simulink model "TST_TClntDspl_DD"  (R2016b)
settings: Solver=FixedStepDiscrete  StartTime=0.0  StopTime=simTime  FixedStep=sampleTime  RelTol=1e-3
values from neighbouring files (symbols this model uses):
  testCase = 1    [initTST_TClntDspl_DD_001.m]    (also in initTST_TClntDspl_DD_002.m = 2; initTST_TClntDspl_DD_003.m = 3; initTST_TClntDspl_DD_004.m = 4; initTST_TClntDspl_DD_005.m = 5)
libraries: simulink x19, UnitTest_Lib x12
settings Model: Creator=liangyunbo  LastModifiedBy=liangyunbo
settings DebuggingCC: SignalRangeChecking=error

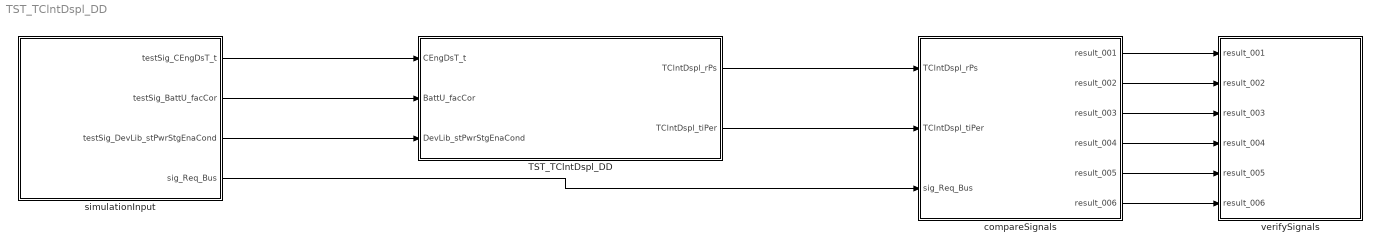
== system TST_TClntDspl_DD ==
  TST_TClntDspl_DD : Subsystem
  compareSignals : Subsystem
  simulationInput : Subsystem
  verifySignals : Subsystem
  wires:
  simulationInput/1(testSig_CEngDsT_t) -> TST_TClntDspl_DD/1(CEngDsT_t)
  simulationInput/2(testSig_BattU_facCor) -> TST_TClntDspl_DD/2(BattU_facCor)
  simulationInput/3(testSig_DevLib_stPwrStgEnaCond) -> TST_TClntDspl_DD/3(DevLib_stPwrStgEnaCond)
  TST_TClntDspl_DD/1(TClntDspl_rPs) -> compareSignals/1(TClntDspl_rPs)
  TST_TClntDspl_DD/2(TClntDspl_tiPer) -> compareSignals/2(TClntDspl_tiPer)
  simulationInput/4(sig_Req_Bus) -> compareSignals/3(sig_Req_Bus)
  compareSignals/1(result_001) -> verifySignals/1(result_001)
  compareSignals/2(result_002) -> verifySignals/2(result_002)
  compareSignals/3(result_003) -> verifySignals/3(result_003)
  compareSignals/4(result_004) -> verifySignals/4(result_004)
  compareSignals/5(result_005) -> verifySignals/5(result_005)
  compareSignals/6(result_006) -> verifySignals/6(result_006)

== system TST_TClntDspl_DD/TST_TClntDspl_DD ==
  CEngDsT_t : Inport
  BattU_facCor : Inport  Port=2
  DevLib_stPwrStgEnaCond : Inport  Port=3
  Function_Call : simulink/Ports & Subsystems/Function-Call Generator  sample_time=sampleTime  numberOfIterations=1
  TClntDspl_DD : ModelReference  ModelNameDialog=TClntDspl_DD  SimulationMode=Normal  ModelReferenceVersion=1.24  TriggerPortName=function  TriggerPortTriggerType=function-call  TriggerPortStatesWhenEnabling=held
  TClntDspl_rPs : Outport
  TClntDspl_tiPer : Outport  Port=2
  wires:
  Function_Call/1 -> TClntDspl_DD/Trigger
  CEngDsT_t/1 -> TClntDspl_DD/1
  BattU_facCor/1 -> TClntDspl_DD/2
  DevLib_stPwrStgEnaCond/1 -> TClntDspl_DD/3
  TClntDspl_DD/1 -> TClntDspl_rPs/1
  TClntDspl_DD/2 -> TClntDspl_tiPer/1

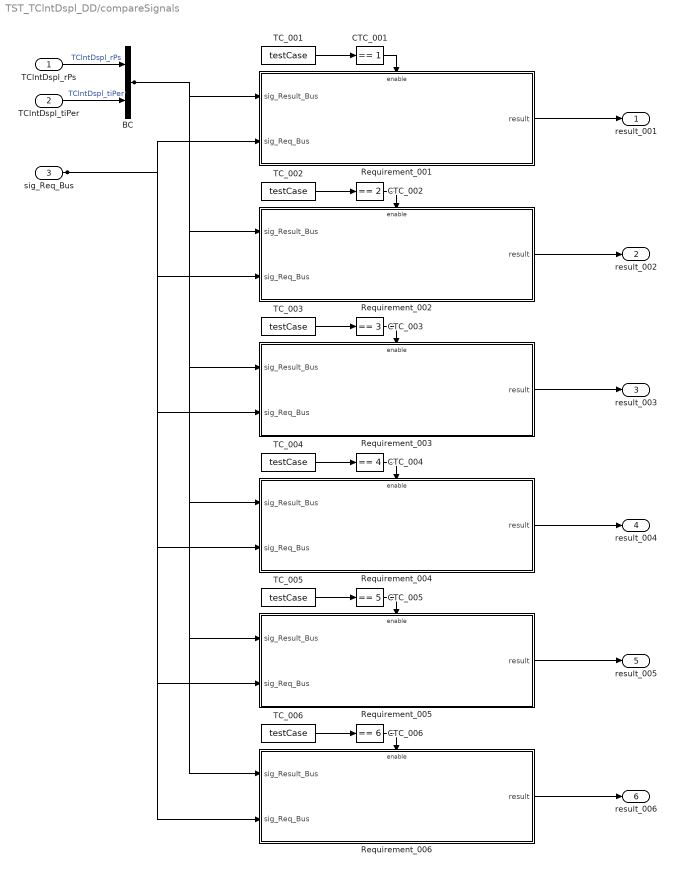
== system TST_TClntDspl_DD/compareSignals ==
  TClntDspl_rPs : Inport
  TClntDspl_tiPer : Inport  Port=2
  sig_Req_Bus : Inport  Port=3
  BC : BusCreator  Inputs=2
  CTC_001 : simulink/Logic and Bit Operations/Compare To Constant  relop===  const=1  OutDataTypeStr=boolean
  CTC_002 : simulink/Logic and Bit Operations/Compare To Constant  relop===  const=2  OutDataTypeStr=boolean
  CTC_003 : simulink/Logic and Bit Operations/Compare To Constant  relop===  const=3  OutDataTypeStr=boolean
  CTC_004 : simulink/Logic and Bit Operations/Compare To Constant  relop===  const=4  OutDataTypeStr=boolean
  CTC_005 : simulink/Logic and Bit Operations/Compare To Constant  relop===  const=5  OutDataTypeStr=boolean
  CTC_006 : simulink/Logic and Bit Operations/Compare To Constant  relop===  const=6  OutDataTypeStr=boolean
  Requirement_001 : Subsystem
  Requirement_002 : Subsystem
  Requirement_003 : Subsystem
  Requirement_004 : Subsystem
  Requirement_005 : Subsystem
  Requirement_006 : Subsystem
  TC_001 : Constant  Value=testCase
  TC_002 : Constant  Value=testCase
  TC_003 : Constant  Value=testCase
  TC_004 : Constant  Value=testCase
  TC_005 : Constant  Value=testCase
  TC_006 : Constant  Value=testCase
  result_001 : Outport
  result_002 : Outport  Port=2
  result_003 : Outport  Port=3
  result_004 : Outport  Port=4
  result_005 : Outport  Port=5
  result_006 : Outport  Port=6
  wires:
  TClntDspl_rPs/1 -> BC/1  "TClntDspl_rPs"
  TClntDspl_tiPer/1 -> BC/2  "TClntDspl_tiPer"
  TC_001/1 -> CTC_001/1
  CTC_001/1 -> Requirement_001/Enable
  sig_Req_Bus/1 -> Requirement_001/2(sig_Req_Bus), Requirement_002/2(sig_Req_Bus), Requirement_003/2(sig_Req_Bus), Requirement_004/2(sig_Req_Bus), Requirement_005/2(sig_Req_Bus), Requirement_006/2(sig_Req_Bus)
  BC/1 -> Requirement_001/1(sig_Result_Bus), Requirement_002/1(sig_Result_Bus), Requirement_003/1(sig_Result_Bus), Requirement_004/1(sig_Result_Bus), Requirement_005/1(sig_Result_Bus), Requirement_006/1(sig_Result_Bus)
  Requirement_001/1(result) -> result_001/1
  TC_002/1 -> CTC_002/1
  CTC_002/1 -> Requirement_002/Enable
  Requirement_002/1(result) -> result_002/1
  TC_003/1 -> CTC_003/1
  CTC_003/1 -> Requirement_003/Enable
  Requirement_003/1(result) -> result_003/1
  TC_004/1 -> CTC_004/1
  CTC_004/1 -> Requirement_004/Enable
  Requirement_004/1(result) -> result_004/1
  TC_005/1 -> CTC_005/1
  CTC_005/1 -> Requirement_005/Enable
  Requirement_005/1(result) -> result_005/1
  TC_006/1 -> CTC_006/1
  CTC_006/1 -> Requirement_006/Enable
  Requirement_006/1(result) -> result_006/1

== system TST_TClntDspl_DD/simulationInput ==
  BS : BusSelector  OutputSignals=testSig_CEngDsT_t,testSig_BattU_facCor,testSig_DevLib_stPwrStgEnaCond
  MPSw : MultiPortSwitch  Inputs=6  SaturateOnIntegerOverflow=on  InputSameDT=on
  TestCase : Constant  Value=testCase
  testSignals_R001 : Subsystem
  testSignals_R002 : Subsystem
  testSignals_R003 : Subsystem
  testSignals_R004 : Subsystem
  testSignals_R005 : Subsystem
  testSignals_R006 : Subsystem
  testSig_CEngDsT_t : Outport
  testSig_BattU_facCor : Outport  Port=2
  testSig_DevLib_stPwrStgEnaCond : Outport  Port=3
  sig_Req_Bus : Outport  Port=4
  wires:
  BS/1 -> testSig_CEngDsT_t/1  "<testSig_CEngDsT_t>"
  BS/2 -> testSig_BattU_facCor/1  "<testSig_BattU_facCor>"
  BS/3 -> testSig_DevLib_stPwrStgEnaCond/1  "<testSig_DevLib_stPwrStgEnaCond>"
  MPSw/1 -> BS/1, sig_Req_Bus/1
  TestCase/1 -> MPSw/1
  testSignals_R001/1(testSignals) -> MPSw/2
  testSignals_R002/1(testSignals) -> MPSw/3
  testSignals_R003/1(testSignals) -> MPSw/4
  testSignals_R004/1(testSignals) -> MPSw/5
  testSignals_R005/1(testSignals) -> MPSw/6
  testSignals_R006/1(testSignals) -> MPSw/7

== system TST_TClntDspl_DD/verifySignals ==
  result_001 : Inport
  result_002 : Inport  Port=2
  result_003 : Inport  Port=3
  result_004 : Inport  Port=4
  result_005 : Inport  Port=5
  result_006 : Inport  Port=6
  Assertion_001 : Assertion  Enabled=off
  Assertion_002 : Assertion  Enabled=off
  Assertion_003 : Assertion  Enabled=off
  Assertion_004 : Assertion  Enabled=off
  Assertion_005 : Assertion  Enabled=off
  Assertion_006 : Assertion  Enabled=off
  wires:
  result_001/1 -> Assertion_001/1
  result_002/1 -> Assertion_002/1
  result_003/1 -> Assertion_003/1
  result_004/1 -> Assertion_004/1
  result_005/1 -> Assertion_005/1
  result_006/1 -> Assertion_006/1

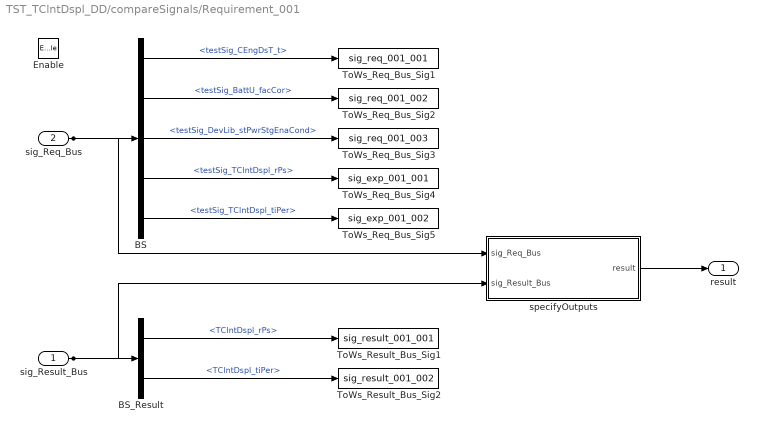
== system TST_TClntDspl_DD/compareSignals/Requirement_001 ==
  sig_Result_Bus : Inport
  sig_Req_Bus : Inport  Port=2
  Enable : EnablePort
  BS : BusSelector  OutputSignals=testSig_CEngDsT_t,testSig_BattU_facCor,testSig_DevLib_stPwrStgEnaCond,testSig_TClntDspl_rPs,testSig_TClntDspl_tiPer
  BS_Result : BusSelector  OutputSignals=TClntDspl_rPs,TClntDspl_tiPer
  ToWs_Req_Bus_Sig1 : ToWorkspace  VariableName=sig_req_001_001  SaveFormat=Structure With Time
  ToWs_Req_Bus_Sig2 : ToWorkspace  VariableName=sig_req_001_002  SaveFormat=Structure With Time
  ToWs_Req_Bus_Sig3 : ToWorkspace  VariableName=sig_req_001_003  SaveFormat=Structure With Time
  ToWs_Req_Bus_Sig4 : ToWorkspace  VariableName=sig_exp_001_001  SaveFormat=Structure With Time
  ToWs_Req_Bus_Sig5 : ToWorkspace  VariableName=sig_exp_001_002  SaveFormat=Structure With Time
  ToWs_Result_Bus_Sig1 : ToWorkspace  VariableName=sig_result_001_001  SaveFormat=Structure With Time
  ToWs_Result_Bus_Sig2 : ToWorkspace  VariableName=sig_result_001_002  SaveFormat=Structure With Time
  specifyOutputs : Subsystem
  result : Outport
  wires:
  sig_Req_Bus/1 -> BS/1, specifyOutputs/1(sig_Req_Bus)
  BS/1 -> ToWs_Req_Bus_Sig1/1  "<testSig_CEngDsT_t>"
  BS/2 -> ToWs_Req_Bus_Sig2/1  "<testSig_BattU_facCor>"
  BS/3 -> ToWs_Req_Bus_Sig3/1  "<testSig_DevLib_stPwrStgEnaCond>"
  BS/4 -> ToWs_Req_Bus_Sig4/1  "<testSig_TClntDspl_rPs>"
  BS/5 -> ToWs_Req_Bus_Sig5/1  "<testSig_TClntDspl_tiPer>"
  sig_Result_Bus/1 -> BS_Result/1, specifyOutputs/2(sig_Result_Bus)
  BS_Result/1 -> ToWs_Result_Bus_Sig1/1  "<TClntDspl_rPs>"
  BS_Result/2 -> ToWs_Result_Bus_Sig2/1  "<TClntDspl_tiPer>"
  specifyOutputs/1(result) -> result/1

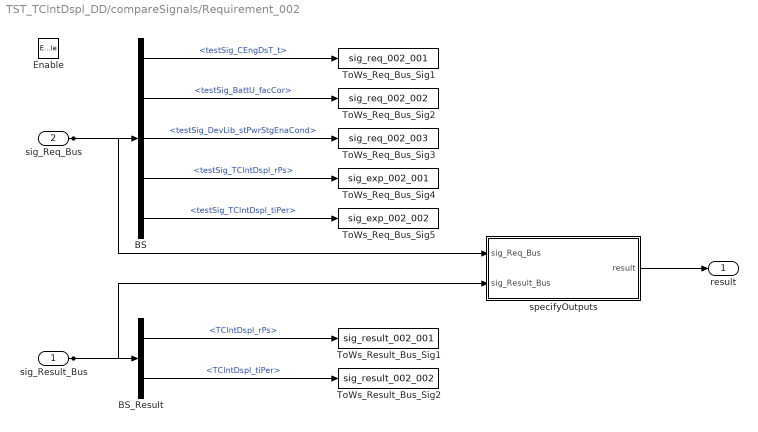
== system TST_TClntDspl_DD/compareSignals/Requirement_002 ==
  sig_Result_Bus : Inport
  sig_Req_Bus : Inport  Port=2
  Enable : EnablePort
  BS : BusSelector  OutputSignals=testSig_CEngDsT_t,testSig_BattU_facCor,testSig_DevLib_stPwrStgEnaCond,testSig_TClntDspl_rPs,testSig_TClntDspl_tiPer
  BS_Result : BusSelector  OutputSignals=TClntDspl_rPs,TClntDspl_tiPer
  ToWs_Req_Bus_Sig1 : ToWorkspace  VariableName=sig_req_002_001  SaveFormat=Structure With Time
  ToWs_Req_Bus_Sig2 : ToWorkspace  VariableName=sig_req_002_002  SaveFormat=Structure With Time
  ToWs_Req_Bus_Sig3 : ToWorkspace  VariableName=sig_req_002_003  SaveFormat=Structure With Time
  ToWs_Req_Bus_Sig4 : ToWorkspace  VariableName=sig_exp_002_001  SaveFormat=Structure With Time
  ToWs_Req_Bus_Sig5 : ToWorkspace  VariableName=sig_exp_002_002  SaveFormat=Structure With Time
  ToWs_Result_Bus_Sig1 : ToWorkspace  VariableName=sig_result_002_001  SaveFormat=Structure With Time
  ToWs_Result_Bus_Sig2 : ToWorkspace  VariableName=sig_result_002_002  SaveFormat=Structure With Time
  specifyOutputs : Subsystem
  result : Outport
  wires:
  sig_Req_Bus/1 -> BS/1, specifyOutputs/1(sig_Req_Bus)
  BS/1 -> ToWs_Req_Bus_Sig1/1  "<testSig_CEngDsT_t>"
  BS/2 -> ToWs_Req_Bus_Sig2/1  "<testSig_BattU_facCor>"
  BS/3 -> ToWs_Req_Bus_Sig3/1  "<testSig_DevLib_stPwrStgEnaCond>"
  BS/4 -> ToWs_Req_Bus_Sig4/1  "<testSig_TClntDspl_rPs>"
  BS/5 -> ToWs_Req_Bus_Sig5/1  "<testSig_TClntDspl_tiPer>"
  sig_Result_Bus/1 -> BS_Result/1, specifyOutputs/2(sig_Result_Bus)
  BS_Result/1 -> ToWs_Result_Bus_Sig1/1  "<TClntDspl_rPs>"
  BS_Result/2 -> ToWs_Result_Bus_Sig2/1  "<TClntDspl_tiPer>"
  specifyOutputs/1(result) -> result/1

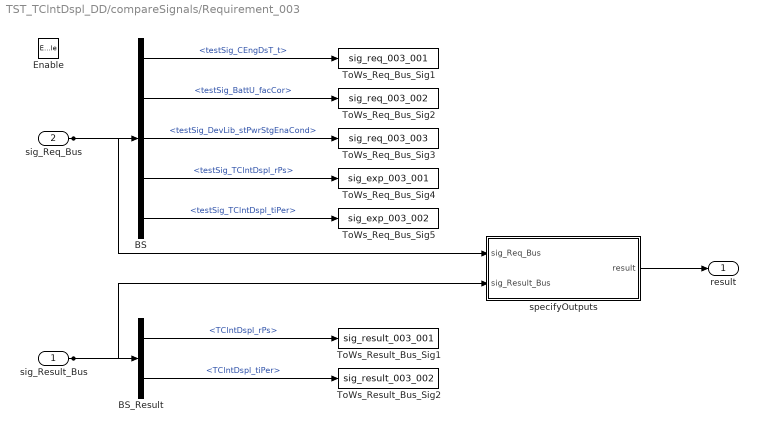
== system TST_TClntDspl_DD/compareSignals/Requirement_003 ==
  sig_Result_Bus : Inport
  sig_Req_Bus : Inport  Port=2
  Enable : EnablePort
  BS : BusSelector  OutputSignals=testSig_CEngDsT_t,testSig_BattU_facCor,testSig_DevLib_stPwrStgEnaCond,testSig_TClntDspl_rPs,testSig_TClntDspl_tiPer
  BS_Result : BusSelector  OutputSignals=TClntDspl_rPs,TClntDspl_tiPer
  ToWs_Req_Bus_Sig1 : ToWorkspace  VariableName=sig_req_003_001  SaveFormat=Structure With Time
  ToWs_Req_Bus_Sig2 : ToWorkspace  VariableName=sig_req_003_002  SaveFormat=Structure With Time
  ToWs_Req_Bus_Sig3 : ToWorkspace  VariableName=sig_req_003_003  SaveFormat=Structure With Time
  ToWs_Req_Bus_Sig4 : ToWorkspace  VariableName=sig_exp_003_001  SaveFormat=Structure With Time
  ToWs_Req_Bus_Sig5 : ToWorkspace  VariableName=sig_exp_003_002  SaveFormat=Structure With Time
  ToWs_Result_Bus_Sig1 : ToWorkspace  VariableName=sig_result_003_001  SaveFormat=Structure With Time
  ToWs_Result_Bus_Sig2 : ToWorkspace  VariableName=sig_result_003_002  SaveFormat=Structure With Time
  specifyOutputs : Subsystem
  result : Outport
  wires:
  sig_Req_Bus/1 -> BS/1, specifyOutputs/1(sig_Req_Bus)
  BS/1 -> ToWs_Req_Bus_Sig1/1  "<testSig_CEngDsT_t>"
  BS/2 -> ToWs_Req_Bus_Sig2/1  "<testSig_BattU_facCor>"
  BS/3 -> ToWs_Req_Bus_Sig3/1  "<testSig_DevLib_stPwrStgEnaCond>"
  BS/4 -> ToWs_Req_Bus_Sig4/1  "<testSig_TClntDspl_rPs>"
  BS/5 -> ToWs_Req_Bus_Sig5/1  "<testSig_TClntDspl_tiPer>"
  sig_Result_Bus/1 -> BS_Result/1, specifyOutputs/2(sig_Result_Bus)
  BS_Result/1 -> ToWs_Result_Bus_Sig1/1  "<TClntDspl_rPs>"
  BS_Result/2 -> ToWs_Result_Bus_Sig2/1  "<TClntDspl_tiPer>"
  specifyOutputs/1(result) -> result/1

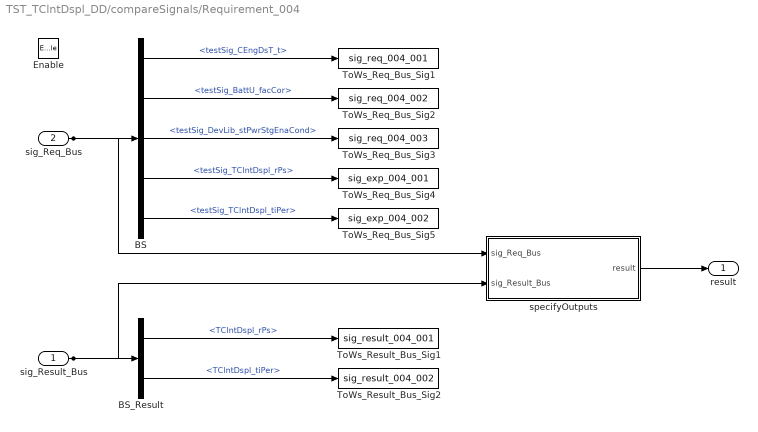
== system TST_TClntDspl_DD/compareSignals/Requirement_004 ==
  sig_Result_Bus : Inport
  sig_Req_Bus : Inport  Port=2
  Enable : EnablePort
  BS : BusSelector  OutputSignals=testSig_CEngDsT_t,testSig_BattU_facCor,testSig_DevLib_stPwrStgEnaCond,testSig_TClntDspl_rPs,testSig_TClntDspl_tiPer
  BS_Result : BusSelector  OutputSignals=TClntDspl_rPs,TClntDspl_tiPer
  ToWs_Req_Bus_Sig1 : ToWorkspace  VariableName=sig_req_004_001  SaveFormat=Structure With Time
  ToWs_Req_Bus_Sig2 : ToWorkspace  VariableName=sig_req_004_002  SaveFormat=Structure With Time
  ToWs_Req_Bus_Sig3 : ToWorkspace  VariableName=sig_req_004_003  SaveFormat=Structure With Time
  ToWs_Req_Bus_Sig4 : ToWorkspace  VariableName=sig_exp_004_001  SaveFormat=Structure With Time
  ToWs_Req_Bus_Sig5 : ToWorkspace  VariableName=sig_exp_004_002  SaveFormat=Structure With Time
  ToWs_Result_Bus_Sig1 : ToWorkspace  VariableName=sig_result_004_001  SaveFormat=Structure With Time
  ToWs_Result_Bus_Sig2 : ToWorkspace  VariableName=sig_result_004_002  SaveFormat=Structure With Time
  specifyOutputs : Subsystem
  result : Outport
  wires:
  sig_Req_Bus/1 -> BS/1, specifyOutputs/1(sig_Req_Bus)
  BS/1 -> ToWs_Req_Bus_Sig1/1  "<testSig_CEngDsT_t>"
  BS/2 -> ToWs_Req_Bus_Sig2/1  "<testSig_BattU_facCor>"
  BS/3 -> ToWs_Req_Bus_Sig3/1  "<testSig_DevLib_stPwrStgEnaCond>"
  BS/4 -> ToWs_Req_Bus_Sig4/1  "<testSig_TClntDspl_rPs>"
  BS/5 -> ToWs_Req_Bus_Sig5/1  "<testSig_TClntDspl_tiPer>"
  sig_Result_Bus/1 -> BS_Result/1, specifyOutputs/2(sig_Result_Bus)
  BS_Result/1 -> ToWs_Result_Bus_Sig1/1  "<TClntDspl_rPs>"
  BS_Result/2 -> ToWs_Result_Bus_Sig2/1  "<TClntDspl_tiPer>"
  specifyOutputs/1(result) -> result/1

== system TST_TClntDspl_DD/compareSignals/Requirement_005 ==
  sig_Result_Bus : Inport
  sig_Req_Bus : Inport  Port=2
  Enable : EnablePort
  BS : BusSelector  OutputSignals=testSig_CEngDsT_t,testSig_BattU_facCor,testSig_DevLib_stPwrStgEnaCond,testSig_TClntDspl_rPs,testSig_TClntDspl_tiPer
  BS_Result : BusSelector  OutputSignals=TClntDspl_rPs,TClntDspl_tiPer
  ToWs_Req_Bus_Sig1 : ToWorkspace  VariableName=sig_req_005_001  SaveFormat=Structure With Time
  ToWs_Req_Bus_Sig2 : ToWorkspace  VariableName=sig_req_005_002  SaveFormat=Structure With Time
  ToWs_Req_Bus_Sig3 : ToWorkspace  VariableName=sig_req_005_003  SaveFormat=Structure With Time
  ToWs_Req_Bus_Sig4 : ToWorkspace  VariableName=sig_exp_005_001  SaveFormat=Structure With Time
  ToWs_Req_Bus_Sig5 : ToWorkspace  VariableName=sig_exp_005_002  SaveFormat=Structure With Time
  ToWs_Result_Bus_Sig1 : ToWorkspace  VariableName=sig_result_005_001  SaveFormat=Structure With Time
  ToWs_Result_Bus_Sig2 : ToWorkspace  VariableName=sig_result_005_002  SaveFormat=Structure With Time
  specifyOutputs : Subsystem
  result : Outport
  wires:
  sig_Req_Bus/1 -> BS/1, specifyOutputs/1(sig_Req_Bus)
  BS/1 -> ToWs_Req_Bus_Sig1/1  "<testSig_CEngDsT_t>"
  BS/2 -> ToWs_Req_Bus_Sig2/1  "<testSig_BattU_facCor>"
  BS/3 -> ToWs_Req_Bus_Sig3/1  "<testSig_DevLib_stPwrStgEnaCond>"
  BS/4 -> ToWs_Req_Bus_Sig4/1  "<testSig_TClntDspl_rPs>"
  BS/5 -> ToWs_Req_Bus_Sig5/1  "<testSig_TClntDspl_tiPer>"
  sig_Result_Bus/1 -> BS_Result/1, specifyOutputs/2(sig_Result_Bus)
  BS_Result/1 -> ToWs_Result_Bus_Sig1/1  "<TClntDspl_rPs>"
  BS_Result/2 -> ToWs_Result_Bus_Sig2/1  "<TClntDspl_tiPer>"
  specifyOutputs/1(result) -> result/1

== system TST_TClntDspl_DD/compareSignals/Requirement_006 ==
  sig_Result_Bus : Inport
  sig_Req_Bus : Inport  Port=2
  Enable : EnablePort
  BS : BusSelector  OutputSignals=testSig_CEngDsT_t,testSig_BattU_facCor,testSig_DevLib_stPwrStgEnaCond,testSig_TClntDspl_rPs,testSig_TClntDspl_tiPer
  BS_Result : BusSelector  OutputSignals=TClntDspl_rPs,TClntDspl_tiPer
  ToWs_Req_Bus_Sig1 : ToWorkspace  VariableName=sig_req_006_001  SaveFormat=Structure With Time
  ToWs_Req_Bus_Sig2 : ToWorkspace  VariableName=sig_req_006_002  SaveFormat=Structure With Time
  ToWs_Req_Bus_Sig3 : ToWorkspace  VariableName=sig_req_006_003  SaveFormat=Structure With Time
  ToWs_Req_Bus_Sig4 : ToWorkspace  VariableName=sig_exp_006_001  SaveFormat=Structure With Time
  ToWs_Req_Bus_Sig5 : ToWorkspace  VariableName=sig_exp_006_002  SaveFormat=Structure With Time
  ToWs_Result_Bus_Sig1 : ToWorkspace  VariableName=sig_result_006_001  SaveFormat=Structure With Time
  ToWs_Result_Bus_Sig2 : ToWorkspace  VariableName=sig_result_006_002  SaveFormat=Structure With Time
  specifyOutputs : Subsystem
  result : Outport
  wires:
  sig_Req_Bus/1 -> BS/1, specifyOutputs/1(sig_Req_Bus)
  BS/1 -> ToWs_Req_Bus_Sig1/1  "<testSig_CEngDsT_t>"
  BS/2 -> ToWs_Req_Bus_Sig2/1  "<testSig_BattU_facCor>"
  BS/3 -> ToWs_Req_Bus_Sig3/1  "<testSig_DevLib_stPwrStgEnaCond>"
  BS/4 -> ToWs_Req_Bus_Sig4/1  "<testSig_TClntDspl_rPs>"
  BS/5 -> ToWs_Req_Bus_Sig5/1  "<testSig_TClntDspl_tiPer>"
  sig_Result_Bus/1 -> BS_Result/1, specifyOutputs/2(sig_Result_Bus)
  BS_Result/1 -> ToWs_Result_Bus_Sig1/1  "<TClntDspl_rPs>"
  BS_Result/2 -> ToWs_Result_Bus_Sig2/1  "<TClntDspl_tiPer>"
  specifyOutputs/1(result) -> result/1

== system TST_TClntDspl_DD/simulationInput/testSignals_R001 ==
  BC : BusCreator  Inputs=5
  spec_BattU_facCor : FromWorkspace  VariableName=testSig_BattU_facCor  Interpolate=off  OutputAfterFinalValue=Holding final value
  spec_CEngDsT_t : FromWorkspace  VariableName=testSig_CEngDsT_t  Interpolate=off  OutputAfterFinalValue=Holding final value
  spec_DevLib_stPwrStgEnaCond : FromWorkspace  VariableName=testSig_DevLib_stPwrStgEnaCond  Interpolate=off  OutputAfterFinalValue=Holding final value
  spec_TClntDspl_rPs : FromWorkspace  VariableName=testSig_TClntDspl_rPs  Interpolate=off  OutputAfterFinalValue=Holding final value
  spec_TClntDspl_tiPer : FromWorkspace  VariableName=testSig_TClntDspl_tiPer  Interpolate=off  OutputAfterFinalValue=Holding final value
  testSignals : Outport
  wires:
  BC/1 -> testSignals/1
  spec_CEngDsT_t/1 -> BC/1  "testSig_CEngDsT_t"
  spec_BattU_facCor/1 -> BC/2  "testSig_BattU_facCor"
  spec_DevLib_stPwrStgEnaCond/1 -> BC/3  "testSig_DevLib_stPwrStgEnaCond"
  spec_TClntDspl_rPs/1 -> BC/4  "testSig_TClntDspl_rPs"
  spec_TClntDspl_tiPer/1 -> BC/5  "testSig_TClntDspl_tiPer"

== system TST_TClntDspl_DD/simulationInput/testSignals_R002 ==
  BC : BusCreator  Inputs=5
  spec_BattU_facCor : FromWorkspace  VariableName=testSig_BattU_facCor  Interpolate=off  OutputAfterFinalValue=Holding final value
  spec_CEngDsT_t : FromWorkspace  VariableName=testSig_CEngDsT_t  Interpolate=off  OutputAfterFinalValue=Holding final value
  spec_DevLib_stPwrStgEnaCond : FromWorkspace  VariableName=testSig_DevLib_stPwrStgEnaCond  Interpolate=off  OutputAfterFinalValue=Holding final value
  spec_TClntDspl_rPs : FromWorkspace  VariableName=testSig_TClntDspl_rPs  Interpolate=off  OutputAfterFinalValue=Holding final value
  spec_TClntDspl_tiPer : FromWorkspace  VariableName=testSig_TClntDspl_tiPer  Interpolate=off  OutputAfterFinalValue=Holding final value
  testSignals : Outport
  wires:
  BC/1 -> testSignals/1
  spec_CEngDsT_t/1 -> BC/1  "testSig_CEngDsT_t"
  spec_BattU_facCor/1 -> BC/2  "testSig_BattU_facCor"
  spec_DevLib_stPwrStgEnaCond/1 -> BC/3  "testSig_DevLib_stPwrStgEnaCond"
  spec_TClntDspl_rPs/1 -> BC/4  "testSig_TClntDspl_rPs"
  spec_TClntDspl_tiPer/1 -> BC/5  "testSig_TClntDspl_tiPer"

== system TST_TClntDspl_DD/simulationInput/testSignals_R003 ==
  BC : BusCreator  Inputs=5
  spec_BattU_facCor : FromWorkspace  VariableName=testSig_BattU_facCor  Interpolate=off  OutputAfterFinalValue=Holding final value
  spec_CEngDsT_t : FromWorkspace  VariableName=testSig_CEngDsT_t  Interpolate=off  OutputAfterFinalValue=Holding final value
  spec_DevLib_stPwrStgEnaCond : FromWorkspace  VariableName=testSig_DevLib_stPwrStgEnaCond  Interpolate=off  OutputAfterFinalValue=Holding final value
  spec_TClntDspl_rPs : FromWorkspace  VariableName=testSig_TClntDspl_rPs  Interpolate=off  OutputAfterFinalValue=Holding final value
  spec_TClntDspl_tiPer : FromWorkspace  VariableName=testSig_TClntDspl_tiPer  Interpolate=off  OutputAfterFinalValue=Holding final value
  testSignals : Outport
  wires:
  BC/1 -> testSignals/1
  spec_CEngDsT_t/1 -> BC/1  "testSig_CEngDsT_t"
  spec_BattU_facCor/1 -> BC/2  "testSig_BattU_facCor"
  spec_DevLib_stPwrStgEnaCond/1 -> BC/3  "testSig_DevLib_stPwrStgEnaCond"
  spec_TClntDspl_rPs/1 -> BC/4  "testSig_TClntDspl_rPs"
  spec_TClntDspl_tiPer/1 -> BC/5  "testSig_TClntDspl_tiPer"

== system TST_TClntDspl_DD/simulationInput/testSignals_R004 ==
  BC : BusCreator  Inputs=5
  spec_BattU_facCor : FromWorkspace  VariableName=testSig_BattU_facCor  Interpolate=off  OutputAfterFinalValue=Holding final value
  spec_CEngDsT_t : FromWorkspace  VariableName=testSig_CEngDsT_t  Interpolate=off  OutputAfterFinalValue=Holding final value
  spec_DevLib_stPwrStgEnaCond : FromWorkspace  VariableName=testSig_DevLib_stPwrStgEnaCond  Interpolate=off  OutputAfterFinalValue=Holding final value
  spec_TClntDspl_rPs : FromWorkspace  VariableName=testSig_TClntDspl_rPs  Interpolate=off  OutputAfterFinalValue=Holding final value
  spec_TClntDspl_tiPer : FromWorkspace  VariableName=testSig_TClntDspl_tiPer  Interpolate=off  OutputAfterFinalValue=Holding final value
  testSignals : Outport
  wires:
  BC/1 -> testSignals/1
  spec_CEngDsT_t/1 -> BC/1  "testSig_CEngDsT_t"
  spec_BattU_facCor/1 -> BC/2  "testSig_BattU_facCor"
  spec_DevLib_stPwrStgEnaCond/1 -> BC/3  "testSig_DevLib_stPwrStgEnaCond"
  spec_TClntDspl_rPs/1 -> BC/4  "testSig_TClntDspl_rPs"
  spec_TClntDspl_tiPer/1 -> BC/5  "testSig_TClntDspl_tiPer"

== system TST_TClntDspl_DD/simulationInput/testSignals_R005 ==
  BC : BusCreator  Inputs=5
  spec_BattU_facCor : FromWorkspace  VariableName=testSig_BattU_facCor  Interpolate=off  OutputAfterFinalValue=Holding final value
  spec_CEngDsT_t : FromWorkspace  VariableName=testSig_CEngDsT_t  Interpolate=off  OutputAfterFinalValue=Holding final value
  spec_DevLib_stPwrStgEnaCond : FromWorkspace  VariableName=testSig_DevLib_stPwrStgEnaCond  Interpolate=off  OutputAfterFinalValue=Holding final value
  spec_TClntDspl_rPs : FromWorkspace  VariableName=testSig_TClntDspl_rPs  Interpolate=off  OutputAfterFinalValue=Holding final value
  spec_TClntDspl_tiPer : FromWorkspace  VariableName=testSig_TClntDspl_tiPer  Interpolate=off  OutputAfterFinalValue=Holding final value
  testSignals : Outport
  wires:
  BC/1 -> testSignals/1
  spec_CEngDsT_t/1 -> BC/1  "testSig_CEngDsT_t"
  spec_BattU_facCor/1 -> BC/2  "testSig_BattU_facCor"
  spec_DevLib_stPwrStgEnaCond/1 -> BC/3  "testSig_DevLib_stPwrStgEnaCond"
  spec_TClntDspl_rPs/1 -> BC/4  "testSig_TClntDspl_rPs"
  spec_TClntDspl_tiPer/1 -> BC/5  "testSig_TClntDspl_tiPer"

== system TST_TClntDspl_DD/simulationInput/testSignals_R006 ==
  BC : BusCreator  Inputs=5
  spec_BattU_facCor : FromWorkspace  VariableName=testSig_BattU_facCor  Interpolate=off  OutputAfterFinalValue=Holding final value
  spec_CEngDsT_t : FromWorkspace  VariableName=testSig_CEngDsT_t  Interpolate=off  OutputAfterFinalValue=Holding final value
  spec_DevLib_stPwrStgEnaCond : FromWorkspace  VariableName=testSig_DevLib_stPwrStgEnaCond  Interpolate=off  OutputAfterFinalValue=Holding final value
  spec_TClntDspl_rPs : FromWorkspace  VariableName=testSig_TClntDspl_rPs  Interpolate=off  OutputAfterFinalValue=Holding final value
  spec_TClntDspl_tiPer : FromWorkspace  VariableName=testSig_TClntDspl_tiPer  Interpolate=off  OutputAfterFinalValue=Holding final value
  testSignals : Outport
  wires:
  BC/1 -> testSignals/1
  spec_CEngDsT_t/1 -> BC/1  "testSig_CEngDsT_t"
  spec_BattU_facCor/1 -> BC/2  "testSig_BattU_facCor"
  spec_DevLib_stPwrStgEnaCond/1 -> BC/3  "testSig_DevLib_stPwrStgEnaCond"
  spec_TClntDspl_rPs/1 -> BC/4  "testSig_TClntDspl_rPs"
  spec_TClntDspl_tiPer/1 -> BC/5  "testSig_TClntDspl_tiPer"

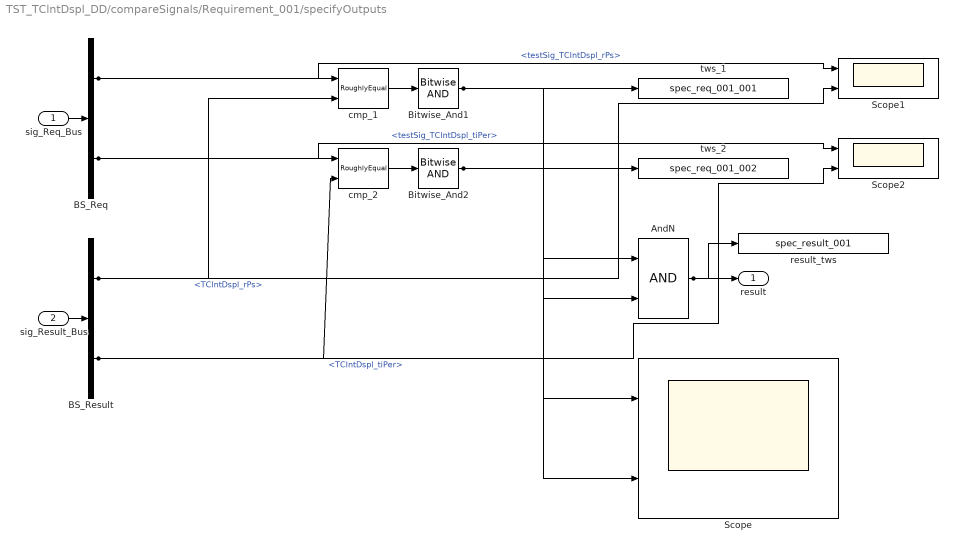
== system TST_TClntDspl_DD/compareSignals/Requirement_001/specifyOutputs ==
  sig_Req_Bus : Inport
  sig_Result_Bus : Inport  Port=2
  AndN : Logic
  BS_Req : BusSelector  OutputSignals=testSig_TClntDspl_rPs,testSig_TClntDspl_tiPer
  BS_Result : BusSelector  OutputSignals=TClntDspl_rPs,TClntDspl_tiPer
  Bitwise_And1 : simulink/Logic and Bit Operations/Bitwise Operator  logicop=AND  UseBitMask=off  BitMask=bin2dec('11011001')  BitMaskRealWorld=Stored Integer
  Bitwise_And2 : simulink/Logic and Bit Operations/Bitwise Operator  logicop=AND  UseBitMask=off  BitMask=bin2dec('11011001')  BitMaskRealWorld=Stored Integer
  Scope : Scope  NumInputPorts=2
  Scope1 : Scope  NumInputPorts=2
  Scope2 : Scope  NumInputPorts=2
  cmp_1 : UnitTest_Lib/RoughlyEqual  slope=0.1
  cmp_2 : UnitTest_Lib/RoughlyEqual  slope=0.1
  result_tws : ToWorkspace  VariableName=spec_result_001
  tws_1 : ToWorkspace  VariableName=spec_req_001_001
  tws_2 : ToWorkspace  VariableName=spec_req_001_002
  result : Outport
  wires:
  sig_Req_Bus/1 -> BS_Req/1
  sig_Result_Bus/1 -> BS_Result/1
  AndN/1 -> result/1, result_tws/1
  BS_Req/1 -> cmp_1/1, Scope1/1  "<testSig_TClntDspl_rPs>"
  BS_Result/1 -> cmp_1/2, Scope1/2  "<TClntDspl_rPs>"
  cmp_1/1 -> Bitwise_And1/1
  Bitwise_And1/1 -> tws_1/1, AndN/1, Scope/1
  BS_Req/2 -> cmp_2/1, Scope2/1  "<testSig_TClntDspl_tiPer>"
  BS_Result/2 -> cmp_2/2, Scope2/2  "<TClntDspl_tiPer>"
  cmp_2/1 -> Bitwise_And2/1
  Bitwise_And2/1 -> tws_2/1, AndN/2, Scope/2

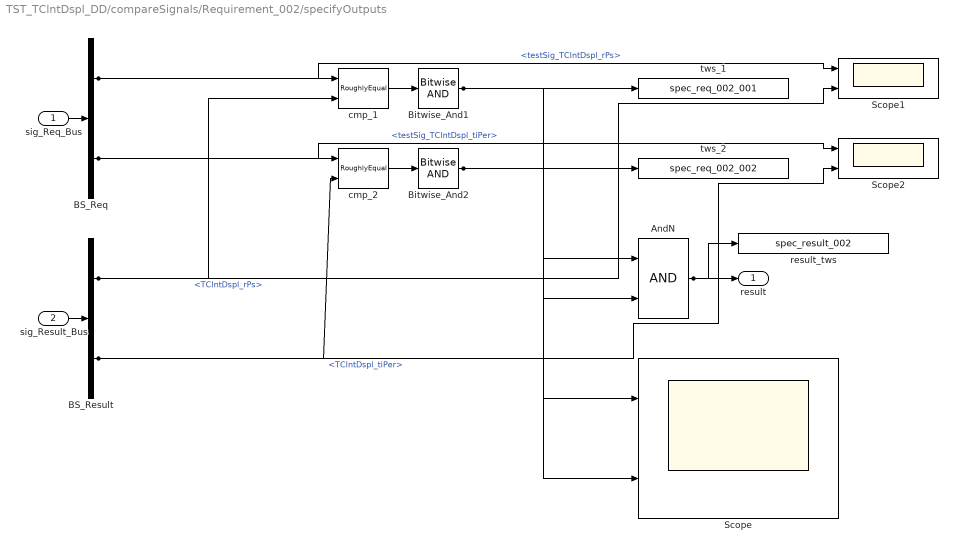
== system TST_TClntDspl_DD/compareSignals/Requirement_002/specifyOutputs ==
  sig_Req_Bus : Inport
  sig_Result_Bus : Inport  Port=2
  AndN : Logic
  BS_Req : BusSelector  OutputSignals=testSig_TClntDspl_rPs,testSig_TClntDspl_tiPer
  BS_Result : BusSelector  OutputSignals=TClntDspl_rPs,TClntDspl_tiPer
  Bitwise_And1 : simulink/Logic and Bit Operations/Bitwise Operator  logicop=AND  UseBitMask=off  BitMask=bin2dec('11011001')  BitMaskRealWorld=Stored Integer
  Bitwise_And2 : simulink/Logic and Bit Operations/Bitwise Operator  logicop=AND  UseBitMask=off  BitMask=bin2dec('11011001')  BitMaskRealWorld=Stored Integer
  Scope : Scope  NumInputPorts=2
  Scope1 : Scope  NumInputPorts=2
  Scope2 : Scope  NumInputPorts=2
  cmp_1 : UnitTest_Lib/RoughlyEqual  slope=0.1
  cmp_2 : UnitTest_Lib/RoughlyEqual  slope=0.1
  result_tws : ToWorkspace  VariableName=spec_result_002
  tws_1 : ToWorkspace  VariableName=spec_req_002_001
  tws_2 : ToWorkspace  VariableName=spec_req_002_002
  result : Outport
  wires:
  sig_Req_Bus/1 -> BS_Req/1
  sig_Result_Bus/1 -> BS_Result/1
  AndN/1 -> result/1, result_tws/1
  BS_Req/1 -> cmp_1/1, Scope1/1  "<testSig_TClntDspl_rPs>"
  BS_Result/1 -> cmp_1/2, Scope1/2  "<TClntDspl_rPs>"
  cmp_1/1 -> Bitwise_And1/1
  Bitwise_And1/1 -> tws_1/1, AndN/1, Scope/1
  BS_Req/2 -> cmp_2/1, Scope2/1  "<testSig_TClntDspl_tiPer>"
  BS_Result/2 -> cmp_2/2, Scope2/2  "<TClntDspl_tiPer>"
  cmp_2/1 -> Bitwise_And2/1
  Bitwise_And2/1 -> tws_2/1, AndN/2, Scope/2

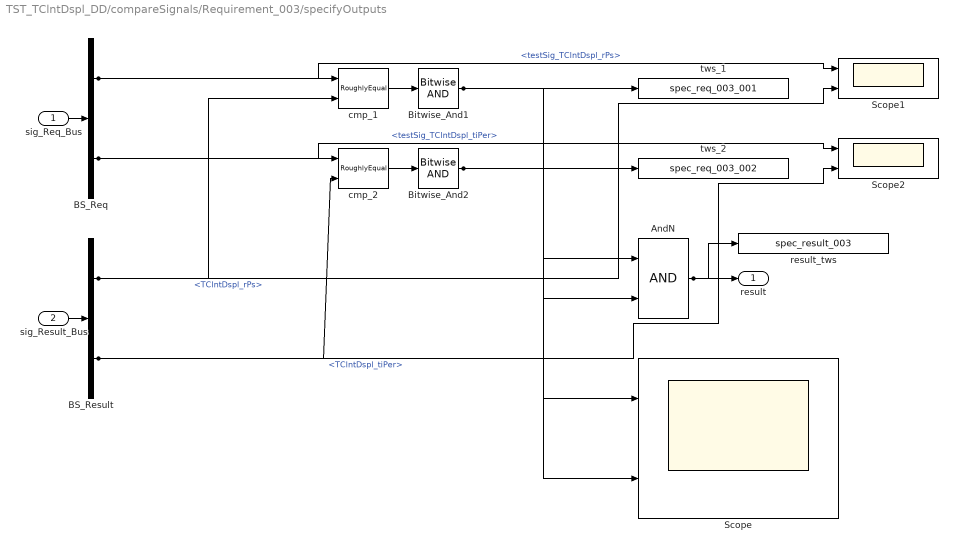
== system TST_TClntDspl_DD/compareSignals/Requirement_003/specifyOutputs ==
  sig_Req_Bus : Inport
  sig_Result_Bus : Inport  Port=2
  AndN : Logic
  BS_Req : BusSelector  OutputSignals=testSig_TClntDspl_rPs,testSig_TClntDspl_tiPer
  BS_Result : BusSelector  OutputSignals=TClntDspl_rPs,TClntDspl_tiPer
  Bitwise_And1 : simulink/Logic and Bit Operations/Bitwise Operator  logicop=AND  UseBitMask=off  BitMask=bin2dec('11011001')  BitMaskRealWorld=Stored Integer
  Bitwise_And2 : simulink/Logic and Bit Operations/Bitwise Operator  logicop=AND  UseBitMask=off  BitMask=bin2dec('11011001')  BitMaskRealWorld=Stored Integer
  Scope : Scope  NumInputPorts=2
  Scope1 : Scope  NumInputPorts=2
  Scope2 : Scope  NumInputPorts=2
  cmp_1 : UnitTest_Lib/RoughlyEqual  slope=0.1
  cmp_2 : UnitTest_Lib/RoughlyEqual  slope=0.1
  result_tws : ToWorkspace  VariableName=spec_result_003
  tws_1 : ToWorkspace  VariableName=spec_req_003_001
  tws_2 : ToWorkspace  VariableName=spec_req_003_002
  result : Outport
  wires:
  sig_Req_Bus/1 -> BS_Req/1
  sig_Result_Bus/1 -> BS_Result/1
  AndN/1 -> result/1, result_tws/1
  BS_Req/1 -> cmp_1/1, Scope1/1  "<testSig_TClntDspl_rPs>"
  BS_Result/1 -> cmp_1/2, Scope1/2  "<TClntDspl_rPs>"
  cmp_1/1 -> Bitwise_And1/1
  Bitwise_And1/1 -> tws_1/1, AndN/1, Scope/1
  BS_Req/2 -> cmp_2/1, Scope2/1  "<testSig_TClntDspl_tiPer>"
  BS_Result/2 -> cmp_2/2, Scope2/2  "<TClntDspl_tiPer>"
  cmp_2/1 -> Bitwise_And2/1
  Bitwise_And2/1 -> tws_2/1, AndN/2, Scope/2

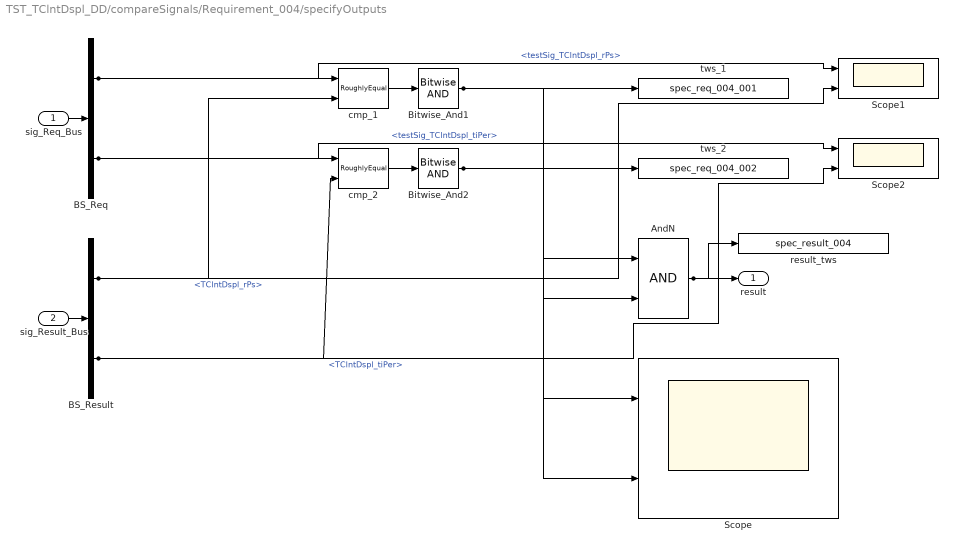
== system TST_TClntDspl_DD/compareSignals/Requirement_004/specifyOutputs ==
  sig_Req_Bus : Inport
  sig_Result_Bus : Inport  Port=2
  AndN : Logic
  BS_Req : BusSelector  OutputSignals=testSig_TClntDspl_rPs,testSig_TClntDspl_tiPer
  BS_Result : BusSelector  OutputSignals=TClntDspl_rPs,TClntDspl_tiPer
  Bitwise_And1 : simulink/Logic and Bit Operations/Bitwise Operator  logicop=AND  UseBitMask=off  BitMask=bin2dec('11011001')  BitMaskRealWorld=Stored Integer
  Bitwise_And2 : simulink/Logic and Bit Operations/Bitwise Operator  logicop=AND  UseBitMask=off  BitMask=bin2dec('11011001')  BitMaskRealWorld=Stored Integer
  Scope : Scope  NumInputPorts=2
  Scope1 : Scope  NumInputPorts=2
  Scope2 : Scope  NumInputPorts=2
  cmp_1 : UnitTest_Lib/RoughlyEqual  slope=0.1
  cmp_2 : UnitTest_Lib/RoughlyEqual  slope=0.1
  result_tws : ToWorkspace  VariableName=spec_result_004
  tws_1 : ToWorkspace  VariableName=spec_req_004_001
  tws_2 : ToWorkspace  VariableName=spec_req_004_002
  result : Outport
  wires:
  sig_Req_Bus/1 -> BS_Req/1
  sig_Result_Bus/1 -> BS_Result/1
  AndN/1 -> result/1, result_tws/1
  BS_Req/1 -> cmp_1/1, Scope1/1  "<testSig_TClntDspl_rPs>"
  BS_Result/1 -> cmp_1/2, Scope1/2  "<TClntDspl_rPs>"
  cmp_1/1 -> Bitwise_And1/1
  Bitwise_And1/1 -> tws_1/1, AndN/1, Scope/1
  BS_Req/2 -> cmp_2/1, Scope2/1  "<testSig_TClntDspl_tiPer>"
  BS_Result/2 -> cmp_2/2, Scope2/2  "<TClntDspl_tiPer>"
  cmp_2/1 -> Bitwise_And2/1
  Bitwise_And2/1 -> tws_2/1, AndN/2, Scope/2

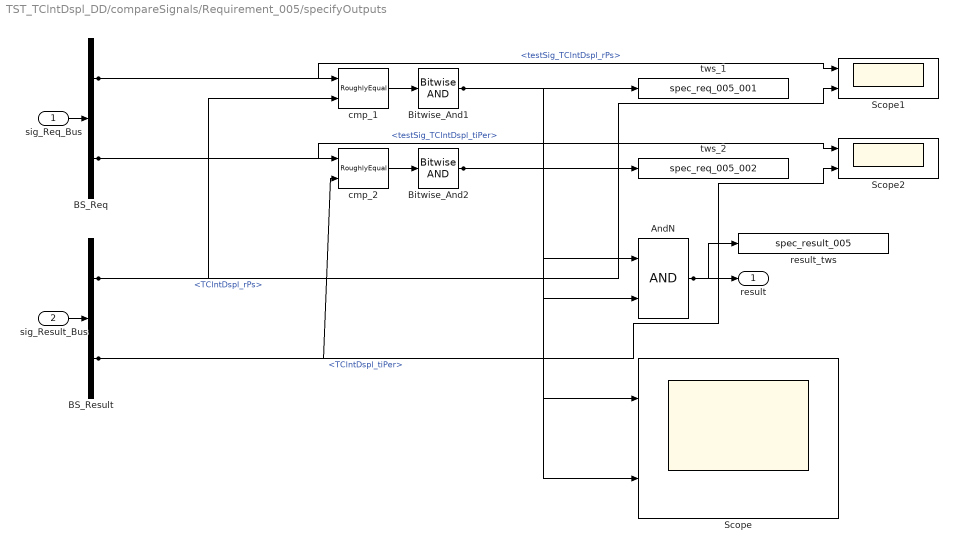
== system TST_TClntDspl_DD/compareSignals/Requirement_005/specifyOutputs ==
  sig_Req_Bus : Inport
  sig_Result_Bus : Inport  Port=2
  AndN : Logic
  BS_Req : BusSelector  OutputSignals=testSig_TClntDspl_rPs,testSig_TClntDspl_tiPer
  BS_Result : BusSelector  OutputSignals=TClntDspl_rPs,TClntDspl_tiPer
  Bitwise_And1 : simulink/Logic and Bit Operations/Bitwise Operator  logicop=AND  UseBitMask=off  BitMask=bin2dec('11011001')  BitMaskRealWorld=Stored Integer
  Bitwise_And2 : simulink/Logic and Bit Operations/Bitwise Operator  logicop=AND  UseBitMask=off  BitMask=bin2dec('11011001')  BitMaskRealWorld=Stored Integer
  Scope : Scope  NumInputPorts=2
  Scope1 : Scope  NumInputPorts=2
  Scope2 : Scope  NumInputPorts=2
  cmp_1 : UnitTest_Lib/RoughlyEqual  slope=0.1
  cmp_2 : UnitTest_Lib/RoughlyEqual  slope=0.1
  result_tws : ToWorkspace  VariableName=spec_result_005
  tws_1 : ToWorkspace  VariableName=spec_req_005_001
  tws_2 : ToWorkspace  VariableName=spec_req_005_002
  result : Outport
  wires:
  sig_Req_Bus/1 -> BS_Req/1
  sig_Result_Bus/1 -> BS_Result/1
  AndN/1 -> result/1, result_tws/1
  BS_Req/1 -> cmp_1/1, Scope1/1  "<testSig_TClntDspl_rPs>"
  BS_Result/1 -> cmp_1/2, Scope1/2  "<TClntDspl_rPs>"
  cmp_1/1 -> Bitwise_And1/1
  Bitwise_And1/1 -> tws_1/1, AndN/1, Scope/1
  BS_Req/2 -> cmp_2/1, Scope2/1  "<testSig_TClntDspl_tiPer>"
  BS_Result/2 -> cmp_2/2, Scope2/2  "<TClntDspl_tiPer>"
  cmp_2/1 -> Bitwise_And2/1
  Bitwise_And2/1 -> tws_2/1, AndN/2, Scope/2

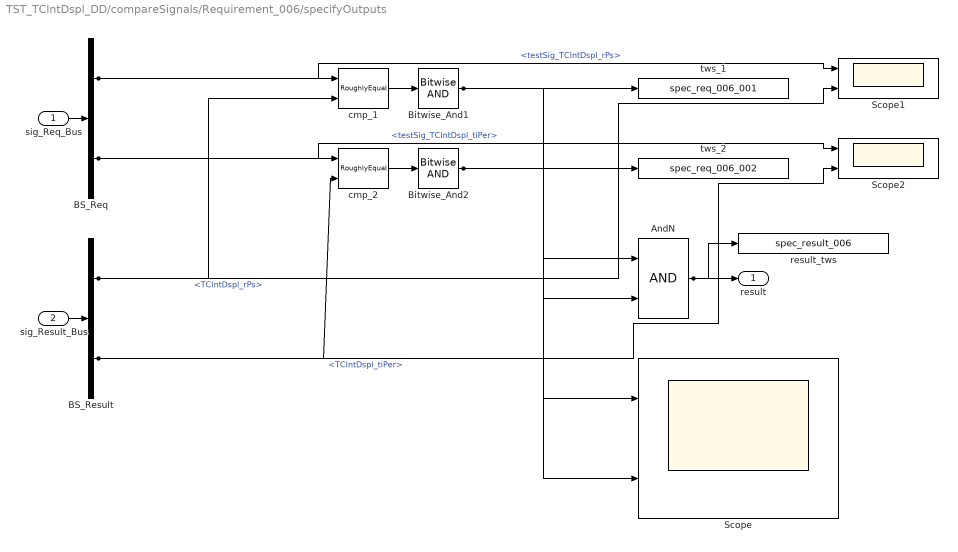
== system TST_TClntDspl_DD/compareSignals/Requirement_006/specifyOutputs ==
  sig_Req_Bus : Inport
  sig_Result_Bus : Inport  Port=2
  AndN : Logic
  BS_Req : BusSelector  OutputSignals=testSig_TClntDspl_rPs,testSig_TClntDspl_tiPer
  BS_Result : BusSelector  OutputSignals=TClntDspl_rPs,TClntDspl_tiPer
  Bitwise_And1 : simulink/Logic and Bit Operations/Bitwise Operator  logicop=AND  UseBitMask=off  BitMask=bin2dec('11011001')  BitMaskRealWorld=Stored Integer
  Bitwise_And2 : simulink/Logic and Bit Operations/Bitwise Operator  logicop=AND  UseBitMask=off  BitMask=bin2dec('11011001')  BitMaskRealWorld=Stored Integer
  Scope : Scope  NumInputPorts=2
  Scope1 : Scope  NumInputPorts=2
  Scope2 : Scope  NumInputPorts=2
  cmp_1 : UnitTest_Lib/RoughlyEqual  slope=0.1
  cmp_2 : UnitTest_Lib/RoughlyEqual  slope=0.1
  result_tws : ToWorkspace  VariableName=spec_result_006
  tws_1 : ToWorkspace  VariableName=spec_req_006_001
  tws_2 : ToWorkspace  VariableName=spec_req_006_002
  result : Outport
  wires:
  sig_Req_Bus/1 -> BS_Req/1
  sig_Result_Bus/1 -> BS_Result/1
  AndN/1 -> result/1, result_tws/1
  BS_Req/1 -> cmp_1/1, Scope1/1  "<testSig_TClntDspl_rPs>"
  BS_Result/1 -> cmp_1/2, Scope1/2  "<TClntDspl_rPs>"
  cmp_1/1 -> Bitwise_And1/1
  Bitwise_And1/1 -> tws_1/1, AndN/1, Scope/1
  BS_Req/2 -> cmp_2/1, Scope2/1  "<testSig_TClntDspl_tiPer>"
  BS_Result/2 -> cmp_2/2, Scope2/2  "<TClntDspl_tiPer>"
  cmp_2/1 -> Bitwise_And2/1
  Bitwise_And2/1 -> tws_2/1, AndN/2, Scope/2
